simulink model "untitled"  (R2014b)
settings: Solver=ode45  StartTime=0.0  StopTime=10.0  RelTol=1e-3
settings Model: Creator=maksimka  LastModifiedBy=maksimka

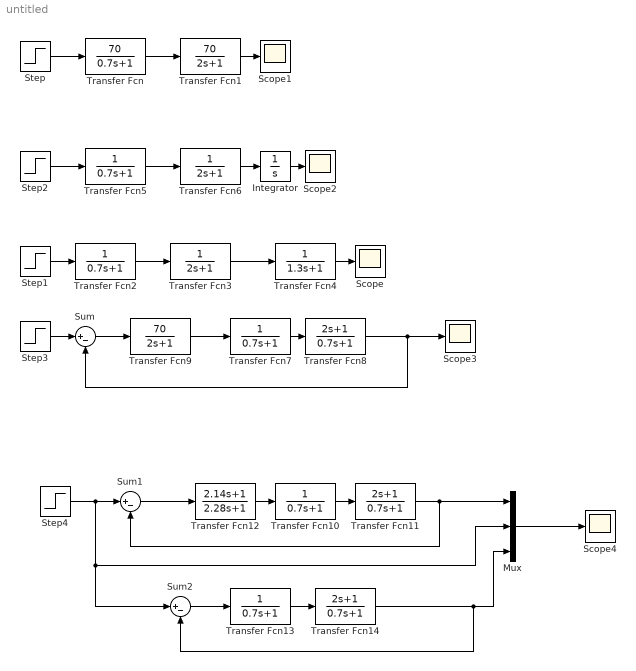
== system untitled ==
  Integrator : Integrator
  Mux : Mux  Inputs=3
  Scope{,1..4} (5 alike) : Scope
      Scope2 settings: SaveName=ScopeData2
      Scope3 settings: SaveName=ScopeData3
      Scope4 settings: SaveName=ScopeData4
  Step{,1..4} (5 alike) : Step  SampleTime=0
  Sum : Sum  Inputs=|+-
  Sum1 : Sum  Inputs=|+-
  Sum2 : Sum  Inputs=|+-
  Transfer Fcn : TransferFcn  Numerator=[70]  Denominator=[0.7 1]
  Transfer Fcn1 : TransferFcn  Numerator=[70]  Denominator=[2 1]
  Transfer Fcn{2,5,7,10,13} (5 alike) : TransferFcn  Denominator=[0.7 1]
  Transfer Fcn11 : TransferFcn  Numerator=[2 1]  Denominator=[0.7 1]
  Transfer Fcn12 : TransferFcn  Numerator=[2.14 1]  Denominator=[2.28 1]
  Transfer Fcn14 : TransferFcn  Numerator=[2 1]  Denominator=[0.7 1]
  Transfer Fcn3 : TransferFcn  Denominator=[2 1]
  Transfer Fcn4 : TransferFcn  Denominator=[1.3 1]
  Transfer Fcn6 : TransferFcn  Denominator=[2 1]
  Transfer Fcn8 : TransferFcn  Numerator=[2 1]  Denominator=[0.7 1]
  Transfer Fcn9 : TransferFcn  Numerator=[70]  Denominator=[2 1]
  wires:
  Step1/1 -> Transfer Fcn2/1
  Step2/1 -> Transfer Fcn5/1
  Transfer Fcn5/1 -> Transfer Fcn6/1
  Step/1 -> Transfer Fcn/1
  Transfer Fcn/1 -> Transfer Fcn1/1
  Transfer Fcn1/1 -> Scope1/1
  Transfer Fcn2/1 -> Transfer Fcn3/1
  Transfer Fcn3/1 -> Transfer Fcn4/1
  Transfer Fcn4/1 -> Scope/1
  Transfer Fcn6/1 -> Integrator/1
  Integrator/1 -> Scope2/1
  Transfer Fcn7/1 -> Transfer Fcn8/1
  Step3/1 -> Sum/1
  Transfer Fcn9/1 -> Transfer Fcn7/1
  Transfer Fcn8/1 -> Scope3/1, Sum/2
  Sum/1 -> Transfer Fcn9/1
  Transfer Fcn10/1 -> Transfer Fcn11/1
  Transfer Fcn12/1 -> Transfer Fcn10/1
  Transfer Fcn11/1 -> Sum1/2, Mux/1
  Sum1/1 -> Transfer Fcn12/1
  Transfer Fcn13/1 -> Transfer Fcn14/1
  Sum2/1 -> Transfer Fcn13/1
  Mux/1 -> Scope4/1
  Step4/1 -> Mux/2, Sum2/1, Sum1/1
  Transfer Fcn14/1 -> Sum2/2, Mux/3
